simulink model "tracking_model2"  (Simulink 8.5)
settings: Solver=ode45  SolverMode=SingleTasking  StartTime=0.0  StopTime=tf  RelTol=1e-5
undefined symbols (not defined in the file or in its folder): sys, x0
settings Model: Creator=brunolnetto  LastModifiedBy=brunolnetto  CovMetricSettings=dwe  CovHtmlReporting=off  covSaveCumulativeToWorkspaceVar=off  CovSaveSingleToWorkspaceVar=off  CovExternalEMLEnable=on
settings DataIOCC: LimitDataPoints=off  SaveFormat=Dataset  SignalLoggingSaveFormat=Dataset
settings OptimizationCC: ExpressionDepthLimit=128
settings DebuggingCC: UnderspecifiedInitializationDetection=Simplified  MergeDetectMultiDrivingBlocksExec=error  FcnCallInpInsideContextMsg=EnableAllAsError  StateNameClashWarn=none  SFUnexpectedBacktrackingDiag=error  SFNoUnconditionalDefaultTransitionDiag=error
settings HardwareCC: ProdBitPerPointer=64  ProdLargestAtomicFloat=Float  ProdIntDivRoundTo=Zero  ProdEndianess=LittleEndian  ProdHWDeviceType=Specified
settings ModelReferenceCC: PropagateSignalLabelsOutOfModel=on
settings GRTTargetCC: TargetLangStandard=C99 (ISO)  GeneratePreprocessorConditionals=Use local settings  CombineOutputUpdateFcns=on  GRTInterface=off

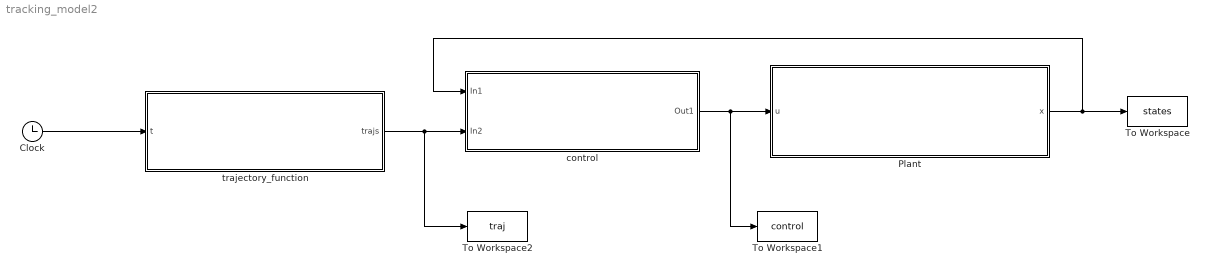
== system tracking_model2 ==
  Clock : Clock
  Plant : Subsystem
      mask Display: image('./plant.png')
  To Workspace : ToWorkspace  VariableName=states  SaveFormat=Structure With Time  SampleTime=-1
  To Workspace1 : ToWorkspace  VariableName=control  SaveFormat=Structure With Time  SampleTime=-1
  To Workspace2 : ToWorkspace  VariableName=traj  SaveFormat=Structure With Time  SampleTime=-1
  control : Subsystem
      mask Display: image('./controller.png');
  trajectory_function : MATLAB Function  TreatAsAtomicUnit=on
      settings: PermitHierarchicalResolution=ParametersOnly
  wires:
  Plant/1(x) -> To Workspace/1, control/1(In1)
  trajectory_function/1(trajs) -> To Workspace2/1, control/2(In2)
  Clock/1 -> trajectory_function/1(t)
  control/1(Out1) -> To Workspace1/1, Plant/1(u)

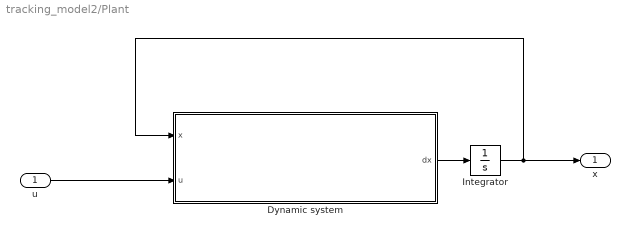
== system tracking_model2/Plant ==
  u : Inport
  Dynamic system : Subsystem
      mask Display: image('./plant.png')
  Integrator : Integrator  InitialCondition=x0
  x : Outport
  wires:
  Dynamic system/1(dx) -> Integrator/1
  u/1 -> Dynamic system/2(u)
  Integrator/1 -> x/1, Dynamic system/1(x)

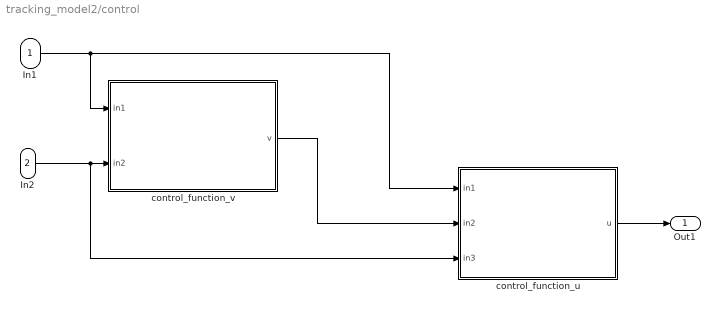
== system tracking_model2/control ==
  In1 : Inport
  In2 : Inport  Port=2
  control_function_u : MATLAB Function  TreatAsAtomicUnit=on
      settings: PermitHierarchicalResolution=ParametersOnly
  control_function_v : MATLAB Function  TreatAsAtomicUnit=on
      settings: PermitHierarchicalResolution=ParametersOnly
  Out1 : Outport
  wires:
  control_function_v/1(v) -> control_function_u/2(in2)
  In1/1 -> control_function_v/1(in1), control_function_u/1(in1)
  control_function_u/1(u) -> Out1/1
  In2/1 -> control_function_u/3(in3), control_function_v/2(in2)

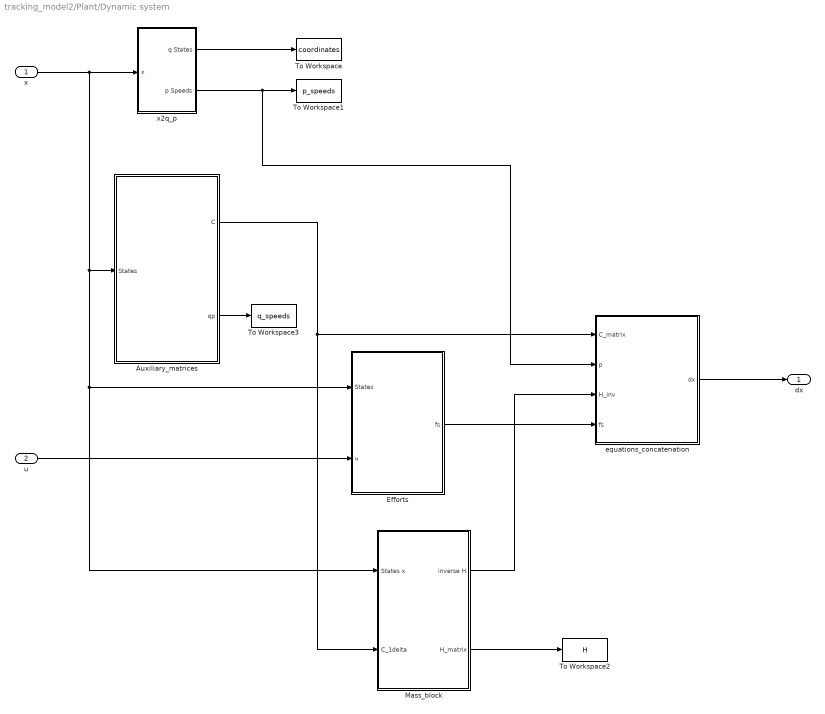
== system tracking_model2/Plant/Dynamic system ==
  x : Inport
  u : Inport  Port=2
  Auxiliary_matrices : Subsystem
  Efforts : Subsystem
  Mass_block : Subsystem
  To Workspace : ToWorkspace  VariableName=coordinates  SaveFormat=Structure With Time  SampleTime=-1
  To Workspace1 : ToWorkspace  VariableName=p_speeds  SaveFormat=Structure With Time  SampleTime=-1
  To Workspace2 : ToWorkspace  VariableName=H  SaveFormat=Structure With Time  SampleTime=-1
  To Workspace3 : ToWorkspace  VariableName=q_speeds  SaveFormat=Structure With Time  SampleTime=-1
  equations_concatenation : Subsystem
  x2q_p : Subsystem
  dx : Outport
  wires:
  Auxiliary_matrices/1(C) -> Mass_block/2("C_1delta  "), equations_concatenation/1(C_matrix)
  Auxiliary_matrices/2(qp) -> To Workspace3/1
  x2q_p/2(p Speeds) -> To Workspace1/1, equations_concatenation/2(p)
  x2q_p/1(q States) -> To Workspace/1
  Efforts/1(fs) -> equations_concatenation/4(fs)
  Mass_block/1(inverse H) -> equations_concatenation/3(H_inv)
  equations_concatenation/1(dx) -> dx/1
  u/1 -> Efforts/2(u)
  x/1 -> x2q_p/1(x), Efforts/1(States), Mass_block/1(States x), Auxiliary_matrices/1(States)
  Mass_block/2(H_matrix) -> To Workspace2/1

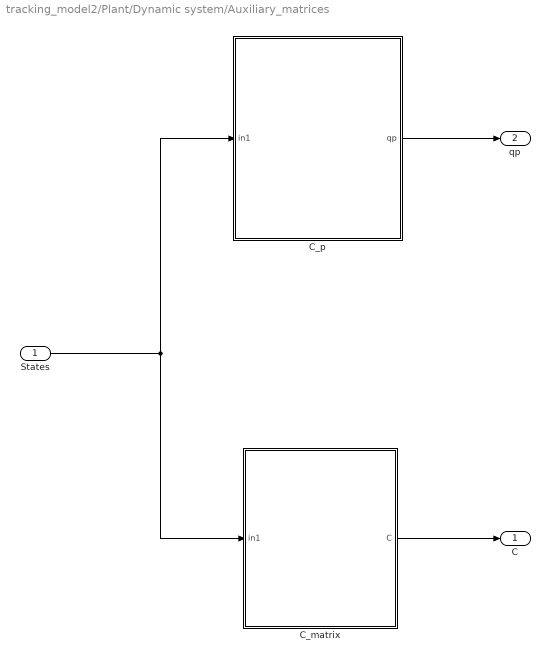
== system tracking_model2/Plant/Dynamic system/Auxiliary_matrices ==
  States : Inport
  C_matrix : MATLAB Function  TreatAsAtomicUnit=on
      settings: PermitHierarchicalResolution=ParametersOnly
  C_p : MATLAB Function  TreatAsAtomicUnit=on
      settings: PermitHierarchicalResolution=ParametersOnly
  C : Outport
  qp : Outport  Port=2
  wires:
  C_matrix/1(C) -> C/1
  States/1 -> C_p/1(in1), C_matrix/1(in1)
  C_p/1(qp) -> qp/1

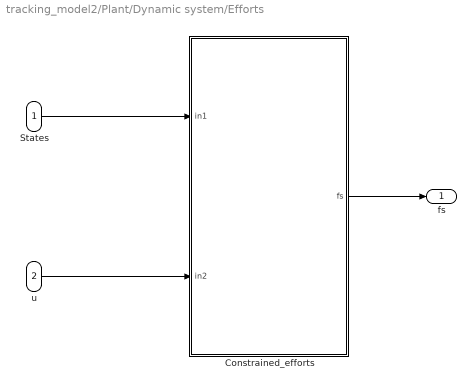
== system tracking_model2/Plant/Dynamic system/Efforts ==
  States : Inport
  u : Inport  Port=2
  Constrained_efforts : MATLAB Function  TreatAsAtomicUnit=on
      settings: PermitHierarchicalResolution=ParametersOnly
  fs : Outport
  wires:
  States/1 -> Constrained_efforts/1(in1)
  u/1 -> Constrained_efforts/2(in2)
  Constrained_efforts/1(fs) -> fs/1

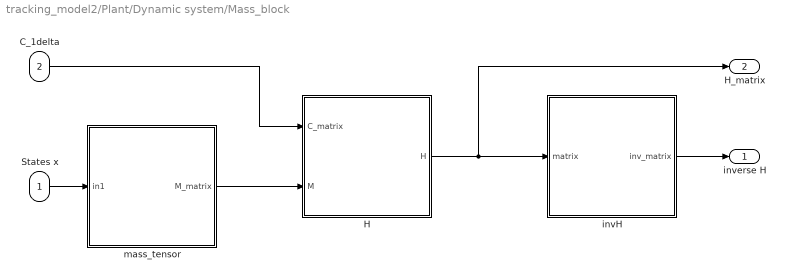
== system tracking_model2/Plant/Dynamic system/Mass_block ==
  States x : Inport
  "C_1delta  " : Inport  Port=2
  H : MATLAB Function  TreatAsAtomicUnit=on
      settings: PermitHierarchicalResolution=ParametersOnly
  invH : MATLAB Function  TreatAsAtomicUnit=on
      settings: PermitHierarchicalResolution=ParametersOnly
  mass_tensor : MATLAB Function  TreatAsAtomicUnit=on
      settings: PermitHierarchicalResolution=ParametersOnly
  inverse H : Outport
  H_matrix : Outport  Port=2
  wires:
  States x/1 -> mass_tensor/1(in1)
  "C_1delta  "/1 -> H/1(C_matrix)
  invH/1(inv_matrix) -> inverse H/1
  H/1(H) -> invH/1(matrix), H_matrix/1
  mass_tensor/1(M_matrix) -> H/2(M)

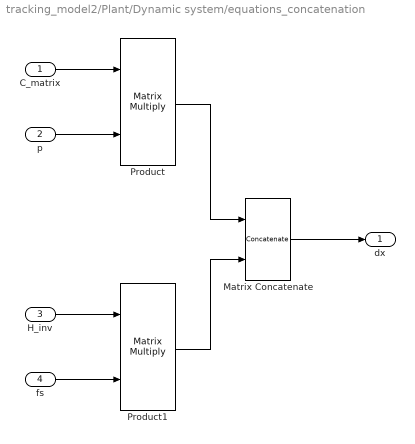
== system tracking_model2/Plant/Dynamic system/equations_concatenation ==
  C_matrix : Inport
  p : Inport  Port=2
  H_inv : Inport  Port=3
  fs : Inport  Port=4
  Matrix Concatenate : Concatenate  ConcatenateDimension=2
  Product : Product  Multiplication=Matrix(*)
  Product1 : Product  Multiplication=Matrix(*)
  dx : Outport
  wires:
  Product/1 -> Matrix Concatenate/1
  p/1 -> Product/2
  C_matrix/1 -> Product/1
  Product1/1 -> Matrix Concatenate/2
  H_inv/1 -> Product1/1
  fs/1 -> Product1/2
  Matrix Concatenate/1 -> dx/1

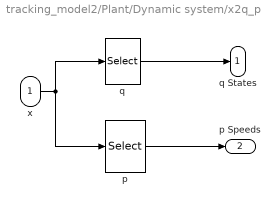
== system tracking_model2/Plant/Dynamic system/x2q_p ==
  x : Inport
  p : Selector  InputPortWidth=length(sys.kin.q) + length(sys.kin.p{end})  IndexOptions=Index vector (dialog)  Indices=(length(sys.kin.q))+1:(length(sys.kin.q) + length(sys.kin.p{end}))  OutputSizes=1
  q : Selector  InputPortWidth=length(sys.kin.q) + length(sys.kin.p{end})  IndexOptions=Index vector (dialog)  Indices=1:length(sys.kin.q)  OutputSizes=1
  q States : Outport
  p Speeds : Outport  Port=2
  wires:
  x/1 -> p/1, q/1
  q/1 -> q States/1
  p/1 -> p Speeds/1

== matlab function control/control_function_u ==
  data: in1 input double; u output double; in2 input double; in3 input double
function u = ControlFunction_u(in1,in2,in3)

%    This function was generated by the Symbolic Math Toolbox version 8.1.

%    14-Sep-2021 12:58:09



p1 = in1(7,:);

p2 = in1(8,:);

p3 = in1(9,:);

phi1 = in1(4,:);

phi2 = in1(5,:);

phi3 = in1(6,:);

th = in1(3,:);

v1 = in2(1,:);

v2 = in2(2,:);

v3 = in2(3,:);

x = in1(1,:);

y = in1(2,:);

y1_ref = in3(1,:);

y2_ref = in3(4,:);

y3_ref = in3(7,:);

yp1_ref = in3(2,:);

yp2_ref = in3(5,:);

yp3_ref = in3(8,:);

ypp1_ref = in3(3,:);

ypp2_ref = in3(6,:);

ypp3_ref = in3(9,:);

t2 = th+5.235987755982989e-1;

t3 = th+1.047197551196598;

t4 = sin(t2);

t5 = sin(t3);

t6 = sin(phi1);

t7 = sin(phi2);

t8 = sin(phi3);

t9 = cos(t2);

t10 = t6.^2;

t11 = t10.*1.862411627770002e-9;

t12 = t7.^2;

t13 = t12.*1.862411627770002e-9;

t14 = t8.^2;

t15 = t14.*1.862411627770002e-9;

t16 = t11+t13+t15-1.044894955682166e-4;

t17 = 1.0./t16;

t18 = cos(t3);

t19 = cos(th);

t20 = sin(th);

t21 = cos(phi1);

t22 = cos(phi2);

t23 = cos(phi3);

t24 = p3.^2;

t25 = t4.*t5.*t17.*1.63236267389886e1;

t26 = t9.*t17.*t19.*1.63236267389886e1;

t27 = t17.*t18.*t20.*-1.63236267389886e1;

t28 = t5.*t17.*t19.*1.63236267389886e1;

t29 = t4.*t17.*t20.*1.63236267389886e1;

t30 = t9.*t17.*t18.*1.63236267389886e1;

t31 = t25+t26+t27+t28+t29+t30;

t32 = 1.0./t31;

t33 = p1.*-2.0e1;

t34 = x.*-1.0e2;

t35 = y1_ref.*1.0e2;

t36 = yp1_ref.*2.0e1;

t37 = t7.*t19.*t22.*t24.*6.008948770734595e-6;

t38 = t8.*t19.*t23.*t24.*-6.008948770734595e-6;

t39 = t6.*t20.*t21.*t24.*6.938536380660578e-6;

t40 = t7.*t20.*t22.*t24.*-3.469268190330289e-6;

t41 = t8.*t20.*t23.*t24.*-3.469268190330289e-6;

t42 = t33+t34+t35+t36+t37+t38+t39+t40+t41+v1+ypp1_ref;

t43 = t5.*t17.*5.924170616113744e-1;

t44 = p2.*-2.0e1;

t45 = y.*-1.0e2;

t46 = y2_ref.*1.0e2;

t47 = yp2_ref.*2.0e1;

t48 = t6.*t19.*t21.*t24.*-6.938536380660578e-6;

t49 = t7.*t19.*t22.*t24.*3.469268190330289e-6;

t50 = t8.*t19.*t23.*t24.*3.469268190330289e-6;

t51 = t7.*t20.*t22.*t24.*6.008948770734595e-6;

t52 = t8.*t20.*t23.*t24.*-6.008948770734595e-6;

t53 = t44+t45+t46+t47+t48+t49+t50+t51+t52+v2+ypp2_ref;

t54 = p3.*-2.0e1;

t55 = th.*-1.0e2;

t56 = y3_ref.*1.0e2;

t57 = yp3_ref.*2.0e1;

t58 = t21.^2;

t59 = t58.*1.164007267356251e62;

t60 = t22.^2;

t61 = t60.*1.164007267356251e62;

t62 = t23.^2;

t63 = t62.*1.164007267356251e62;

t64 = t59+t61+t63+6.530244270833333e66;

t65 = 1.0./t64;

t66 = phi1.*2.0;

t67 = sin(t66);

t68 = t24.*t67.*1.691871028134086e62;

t69 = phi2.*2.0;

t70 = sin(t69);

t71 = t24.*t70.*1.691871028134086e62;

t72 = phi3.*2.0;

t73 = sin(t72);

t74 = t24.*t73.*1.691871028134086e62;

t75 = t24.*3.926713624160408e26;

t76 = p2.*p3.*t6.*t19.*t21.*2.706993645014537e63;

t77 = p1.*p3.*t7.*t19.*t22.*-2.344325264465624e63;

t78 = p2.*p3.*t7.*t19.*t22.*-1.353496822507269e63;

t79 = p1.*p3.*t8.*t19.*t23.*2.344325264465624e63;

t80 = p2.*p3.*t8.*t19.*t23.*-1.353496822507269e63;

t81 = p1.*p3.*t6.*t20.*t21.*-2.706993645014537e63;

t82 = p1.*p3.*t7.*t20.*t22.*1.353496822507269e63;

t83 = p2.*p3.*t7.*t20.*t22.*-2.344325264465624e63;

t84 = p1.*p3.*t8.*t20.*t23.*1.353496822507269e63;

t85 = p2.*p3.*t8.*t20.*t23.*2.344325264465624e63;

t86 = t68+t71+t74+t75+t76+t77+t78+t79+t80+t81+t82+t83+t84+t85;

t87 = t65.*t86.*1.0;

t88 = t54+t55+t56+t57+t87+v3+ypp3_ref;

t89 = t9.*t17.*5.924170616113744e-1;

t90 = t4.*t17.*5.924170616113744e-1;

t91 = t17.*t19.*5.924170616113744e-1;

u = [t32.*t53.*(t43+t89).*-1.0+t32.*t42.*(t90-t17.*t18.*5.924170616113744e-1).*1.0+t32.*t88.*(t4.*t5.*7.592384529762141e2+t9.*t18.*7.592384529762141e2);t32.*t53.*(t43+t17.*t20.*5.924170616113744e-1)+t32.*t42.*(t91+t17.*t18.*5.924170616113744e-1)+t32.*t88.*(t5.*t19.*7.592384529762141e2-t18.*t20.*7.592384529762141e2);t32.*t42.*(t90+t91).*-1.0+t32.*t53.*(t89-t17.*t20.*5.924170616113744e-1)+t32.*t88.*(t4.*t20.*7.592384529762141e2+t9.*t19.*7.592384529762141e2)];

end

== matlab function Plant/Dynamic system/Mass_block/mass_tensor ==
  data: in1 input double; M_matrix output double
function M_matrix = Mass_matrix(in1)

%    This function was generated by the Symbolic Math Toolbox version 8.1.

%    14-Sep-2021 12:58:16



phi1 = in1(4,:);

phi2 = in1(5,:);

phi3 = in1(6,:);

th = in1(3,:);

t2 = cos(phi1);

t3 = cos(phi2);

t4 = cos(phi3);

t5 = cos(th);

t6 = sin(th);

t8 = t5.*(1.0./8.0);

t9 = sqrt(3.0);

t10 = t6.*t9.*(1.0./8.0);

t7 = t8-t10;

t11 = t8+t10;

t13 = t6.*(1.0./8.0);

t14 = t5.*t9.*(1.0./8.0);

t12 = t13-t14;

t15 = t13+t14;

M_matrix = reshape([2.11e2./5.0e2,0.0,0.0,0.0,0.0,0.0,0.0,2.11e2./5.0e2,0.0,0.0,0.0,0.0,0.0,0.0,t2.^2.*2.518133623269337e-7+t3.^2.*2.518133623269337e-7+t4.^2.*2.518133623269337e-7+t5.^2.*4.625e-3+t6.^2.*4.625e-3+t7.^2.*(3.7e1./5.0e2)+t11.^2.*(3.7e1./5.0e2)+t12.^2.*(3.7e1./5.0e2)+t15.^2.*(3.7e1./5.0e2)+2.520833333333333e-4,0.0,0.0,0.0,0.0,0.0,0.0,0.0,0.0,0.0,0.0,0.0,0.0,0.0,0.0,0.0,0.0,0.0,0.0,0.0,0.0,0.0],[6,6]);

end

== matlab function Plant/Dynamic system/Auxiliary_matrices/C_matrix ==
  data: in1 input double; C output double
function C = ConstraintMatrix(in1)

%    This function was generated by the Symbolic Math Toolbox version 8.1.

%    14-Sep-2021 12:58:16



th = in1(3,:);

t2 = pi.*(1.0./3.0);

t3 = t2+th;

C = reshape([1.0,0.0,0.0,sin(th).*(5.0e2./4.3e1),cos(th+pi.*(1.0./6.0)).*(5.0e2./4.3e1),sin(t3).*(-5.0e2./4.3e1),0.0,1.0,0.0,cos(th).*(-5.0e2./4.3e1),cos(th-pi.*(1.0./3.0)).*(5.0e2./4.3e1),cos(t3).*(5.0e2./4.3e1),0.0,0.0,1.0,-1.25e2./4.3e1,-1.25e2./4.3e1,-1.25e2./4.3e1],[6,3]);

end

== matlab function trajectory_function ==
  data: t input double; trajs output double
function trajs = TrajectoryGenerator(t)

%    This function was generated by the Symbolic Math Toolbox version 8.1.

%    14-Sep-2021 12:58:13



t2 = cos(t);

t3 = sin(t);

trajs = [t2;-t3;-t2;t3;t2;-t3;t;1.0;0.0];

end

== matlab function control/control_function_v ==
  data: in1 input double; v output double; in2 input double
function v = ControlFunction_v(in1,in2)

%    This function was generated by the Symbolic Math Toolbox version 8.1.

%    14-Sep-2021 12:58:10



p1 = in1(7,:);

p2 = in1(8,:);

p3 = in1(9,:);

th = in1(3,:);

x = in1(1,:);

y = in1(2,:);

y1_ref = in2(1,:);

y2_ref = in2(4,:);

y3_ref = in2(7,:);

yp1_ref = in2(2,:);

yp2_ref = in2(5,:);

yp3_ref = in2(8,:);

v = [p1.*-1.002179860514571e1-p2.*5.838405801408701e-1-p3.*8.693126705171474e-14-th.*1.323367093602647e-12-x.*1.081952593981158e2-y.*1.122253116268095e1+y1_ref.*1.081952593981158e2+y2_ref.*1.122253116268095e1+y3_ref.*1.323367093602647e-12+yp1_ref.*1.002179860514571e1+yp2_ref.*5.838405801408701e-1+yp3_ref.*8.693126705171474e-14;p1.*-6.112050255810735e-1-p2.*4.933703568966422-p3.*9.004259724936276e-13-th.*8.941284373818785e-12-x.*1.163592064118006e1-y.*8.766593630617706+y1_ref.*1.163592064118006e1+y2_ref.*8.766593630617706+y3_ref.*8.941284373818785e-12+yp1_ref.*6.112050255810735e-1+yp2_ref.*4.933703568966422+yp3_ref.*9.004259724936276e-13;p1.*-5.136251536432802e-14-p2.*7.215305464827268e-13+p3.*5.402006975503619+th.*7.53277692072209e1-x.*7.460358889351478e-13-y.*6.695044661662565e-12+y1_ref.*7.460358889351478e-13+y2_ref.*6.695044661662565e-12-y3_ref.*7.53277692072209e1+yp1_ref.*5.136251536432802e-14+yp2_ref.*7.215305464827268e-13-yp3_ref.*5.402006975503619];

end

== matlab function Plant/Dynamic system/Efforts/Constrained_efforts ==
  data: in1 input double; fs output double; in2 input double
function fs = ConstrainedEffort(in1,in2)

%    This function was generated by the Symbolic Math Toolbox version 8.1.

%    14-Sep-2021 12:58:16



p1 = in1(7,:);

p2 = in1(8,:);

p3 = in1(9,:);

phi1 = in1(4,:);

phi2 = in1(5,:);

phi3 = in1(6,:);

tau1 = in2(1,:);

tau2 = in2(2,:);

tau3 = in2(3,:);

th = in1(3,:);

t2 = sin(th);

t3 = sqrt(3.0);

t4 = cos(th);

t5 = p3.^2;

t6 = t2.*t3;

t7 = cos(phi2);

t8 = sin(phi2);

t9 = th+1.047197551196598;

t10 = cos(phi3);

t11 = sin(phi3);

t12 = cos(phi1);

t13 = sin(phi1);

t14 = p3.*t2.*1.25e-1;

t36 = p3.*t4.*2.165063509461097e-1;

t35 = -t36;

t33 = -t35;

t28 = -t33;

t17 = -t28;

t15 = -t17;

t16 = t14+t15;

t18 = t4.*1.25e-1;

t37 = p3.*t4.*-1.25e-1;

t31 = -t37;

t30 = -t31;

t19 = -t30;

t34 = p3.*t2.*2.165063509461097e-1;

t32 = -t34;

t20 = -t32;

t21 = t4.*2.165063509461097e-1;

t22 = p2.*-1.0;

t23 = t19+t20+t22;

t24 = t2.*1.25e-1;

t25 = t21-t24;

t26 = t2.*2.165063509461097e-1;

t27 = t18+t26;

t29 = t21+t24;

t38 = p3.*t4.*(1.0./4.0);

t39 = p2+t38;

t40 = p3.*t2.*-2.5e-1;

t41 = p1+t40;

t42 = th+5.235987755982989e-1;

t43 = cos(t42);

t44 = th-1.047197551196598;

t45 = cos(t44);

t46 = p3.*(1.25e2./4.3e1);

t47 = cos(t9);

t48 = sin(t9);

fs = [t2.*tau1.*(5.0e2./4.3e1)-tau2.*(t2-t3.*t4).*(2.5e2./4.3e1)-tau3.*(t2+t3.*t4).*(2.5e2./4.3e1)-t2.*t5.*t12.*t13.*2.928062352638764e-6-t5.*t7.*t8.*t43.*2.928062352638764e-6+t5.*t10.*t11.*t48.*2.928062352638764e-6;tau2.*(t4+t6).*(2.5e2./4.3e1)-t4.*tau1.*(5.0e2./4.3e1)+tau3.*(t4-t6).*(2.5e2./4.3e1)+t4.*t5.*t12.*t13.*2.928062352638764e-6-t5.*t7.*t8.*t45.*2.928062352638764e-6-t5.*t10.*t11.*t47.*2.928062352638764e-6;tau1.*(-1.25e2./4.3e1)-tau2.*(1.25e2./4.3e1)-tau3.*(1.25e2./4.3e1)-t16.*t23.*(3.7e1./5.0e2)+p3.*(t25.*(t19+t20).*7.4e-2+t2.*t39.*1.85e-2+t16.*t27.*(3.7e1./5.0e2)+t4.*t41.*1.85e-2-t23.*t25.*(3.7e1./5.0e2)+(t14+t17).*(t18-t26).*(3.7e1./5.0e2)-t29.*(t19-p3.*t2.*2.165063509461097e-1).*7.4e-2-t27.*(p1+t14+t28).*7.4e-2-t29.*(p2+t20+t30).*7.4e-2-(t18-t26).*(p1+t14+t17).*7.4e-2).*1.0+(t31+t32).*(p1+t14+t33).*7.4e-2+(t31+t34).*(p1+t14+t35).*7.4e-2+(t14+t36).*(p2+t34+t37).*7.4e-2-p3.*t2.*t39.*1.85e-2-p3.*t4.*t41.*1.85e-2+t5.*t7.*t8.*7.32015588159691e-7+t5.*t10.*t11.*7.32015588159691e-7+t5.*t12.*t13.*7.32015588159691e-7-p3.*t12.*t13.*(t46-p1.*t2.*1.162790697674419e1+p2.*t4.*(5.0e2./4.3e1)).*5.036267246538674e-7-p3.*t10.*t11.*(t46+p1.*t48.*(5.0e2./4.3e1)-p2.*t47.*1.162790697674419e1).*5.036267246538674e-7+p3.*t7.*t8.*(p3.*-2.906976744186047+p1.*t43.*(5.0e2./4.3e1)+p2.*t45.*(5.0e2./4.3e1)).*5.036267246538674e-7];

end

== matlab function Plant/Dynamic system/Mass_block/H ==
  data: C_matrix input double; H output double; M input double
function H = ConstrinedMassMatrix(C_matrix, M)
% MASSMATRIX
%    This function was generated by the Symbolic Math Toolbox version 7.2.
%    16-Oct-2020 11:55:07

    H = C_matrix'*M*C_matrix;
end

== matlab function Plant/Dynamic system/Mass_block/invH ==
  data: matrix input double; inv_matrix output double
function inv_matrix = matrix_inverse(matrix)
% MASSMATRIX
%    This function was generated by the Symbolic Math Toolbox version 7.2.
%    16-Oct-2020 11:55:07

    inv_matrix = inv(matrix);
end

== matlab function Plant/Dynamic system/Auxiliary_matrices/C_p ==
  data: in1 input double; qp output double
function qp = KinematicVector(in1)

%    This function was generated by the Symbolic Math Toolbox version 8.1.

%    14-Sep-2021 12:58:15



p1 = in1(7,:);

p2 = in1(8,:);

p3 = in1(9,:);

th = in1(3,:);

t2 = pi.*(1.0./3.0);

t3 = t2+th;

qp = [p1;p2;p3;p3.*(-1.25e2./4.3e1)-p2.*cos(th).*(5.0e2./4.3e1)+p1.*sin(th).*(5.0e2./4.3e1);p3.*(-1.25e2./4.3e1)+p2.*cos(th-pi.*(1.0./3.0)).*(5.0e2./4.3e1)+p1.*cos(th+pi.*(1.0./6.0)).*(5.0e2./4.3e1);p3.*(-1.25e2./4.3e1)+p2.*cos(t3).*(5.0e2./4.3e1)-p1.*sin(t3).*(5.0e2./4.3e1)];

end
